simulink library "motor3D_cl"  (R2020a)
settings: Solver=VariableStepAuto  StartTime=0.0  StopTime=10.0  RelTol=1e-3
undefined symbols (not defined in the file): Veh
libraries: simulink x2, vrlib x1, thrustCurve_ul x1
settings Model: Creator=John Jr  LastModifiedBy=John Jr

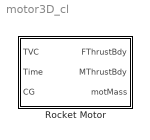
== system motor3D_cl ==
  Rocket Motor : Subsystem  mask{m_m=Veh.motor.motorMass.Value, m_f=Veh.motor.fuelMass.Value, t_b=Veh.motor.burnTime.Value, rM=Veh.motor.position.Value}
      mask prompts: m_m "Total motor mass [kg]"; m_f "Propellant mass [kg]"; t_b "Motor burn time [s]"; rM "Motor position [m]"
      mask DialogControl DescGroupVar Prompt: Rocket Motor Library
      mask DialogControl DescTextVar Prompt: This block models the motor's thrust acting on the vehicle, including rotational effects.
      mask Display:
      | patch([0 1 1 0], [0 0 1 1],[.8 1 1])
      | 
      | port_label('input',1,'\fontname{Cambria Math}Control','texmode','on')
      | port_label('input',2,'\fontname{Cambria Math}Time','texmode','on')
      | port_label('input',3,'\fontname{Cambria Math}rCM_B','texmode','on')
      | 
      | port_label('output',1,'\fontname{Cambria Math}FThrustBdy','texmode','on')
      | port_label('output',2,'\fontname{Cambria Math}MThrustBdy','texmode','on')
      | port_label('output',3,'\fontname{Cambria Math}motorMass','texmode','on')

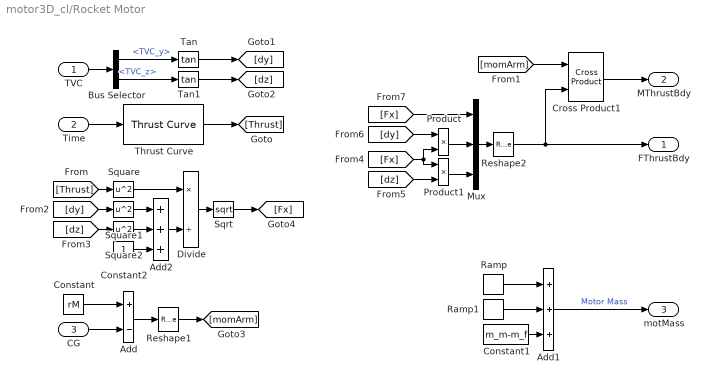
== system motor3D_cl/Rocket Motor ==
  TVC : Inport
  Time : Inport  Port=2
  CG : Inport  Port=3
  Add : Sum  Inputs=+-
  Add1 : Sum  Inputs=+++
  Add2 : Sum  Inputs=+++
  Bus Selector : BusSelector  OutputSignals=TVC_y,TVC_z
  Constant : Constant  Value=rM
  Constant1 : Constant  Value=m_m-m_f
  Constant2 : Constant
  Cross Product1 : vrlib/Utilities/Cross Product
  Divide : Product  Inputs=*/
  Mux : Mux  Inputs=3
  Product : Product
  Product1 : Product
  Ramp : simulink/Sources/Ramp  slope=-m_f/t_b  start=0  InitialOutput=m_f
  Ramp1 : simulink/Sources/Ramp  slope=m_f/t_b  start=t_b  InitialOutput=0
  Reshape1 : Reshape  OutputDimensionality=Column vector (2-D)
  Reshape2 : Reshape  OutputDimensionality=Column vector (2-D)
  Sqrt : Sqrt  SaturateOnIntegerOverflow=on
  Square : Math  Operator=square  SaturateOnIntegerOverflow=on
  Square1 : Math  Operator=square  SaturateOnIntegerOverflow=on
  Square2 : Math  Operator=square  SaturateOnIntegerOverflow=on
  Tan : Trigonometry  Operator=tan
  Tan1 : Trigonometry  Operator=tan
  "Thrust Curve " : thrustCurve_ul/Thrust Curve   F_th=Veh.motor.thrustVec.Value  T_b=Veh.motor.burnTimeVec.Value  eta=Veh.motor.efficiency.Value
  FThrustBdy : Outport  VectorParamsAs1DForOutWhenUnconnected=off
  MThrustBdy : Outport  Port=2  VectorParamsAs1DForOutWhenUnconnected=off
  motMass : Outport  Port=3  VectorParamsAs1DForOutWhenUnconnected=off
  wires:
  Bus Selector/2 -> Tan1/1  "<TVC_z>"
  Bus Selector/1 -> Tan/1  "<TVC_y>"
  [Fx] -> Mux/1
  Product1/1 -> Mux/3
  Product/1 -> Mux/2
  "Thrust Curve "/1 -> [Thrust]
  Ramp/1 -> Add1/1
  Constant1/1 -> Add1/3
  Ramp1/1 -> Add1/2
  Time/1 -> "Thrust Curve "/1
  Constant/1 -> Add/1
  CG/1 -> Add/2
  Add1/1 -> motMass/1  "Motor Mass"
  Add/1 -> Reshape1/1
  Reshape1/1 -> [momArm]
  Cross Product1/1 -> MThrustBdy/1
  [momArm] -> Cross Product1/1
  TVC/1 -> Bus Selector/1
  [Thrust] -> Square/1
  [dy] -> Square1/1
  [dz] -> Square2/1
  Square1/1 -> Add2/1
  Square2/1 -> Add2/2
  Constant2/1 -> Add2/3
  Add2/1 -> Divide/2
  Square/1 -> Divide/1
  Divide/1 -> Sqrt/1
  Tan/1 -> [dy]
  Tan1/1 -> [dz]
  Sqrt/1 -> [Fx]
  [dy] -> Product/1
  [Fx] -> Product/2, Product1/1
  [dz] -> Product1/2
  Mux/1 -> Reshape2/1
  Reshape2/1 -> Cross Product1/2, FThrustBdy/1
